simulink model "FM_Broadcast_CE2251"  (R2025a)
settings: Solver=FixedStepDiscrete  StartTime=0.0  StopTime=inf  RelTol=1e-3  EnableMultiTasking=on
PostLoadFcn:
  | blk = [gcs,'/Spectrum Analyzer'];
  | cfg = get_param(blk,'ScopeConfiguration');
libraries: dspsnks4 x1, dspsigops x1, commanabbnd3 x1, sdrrlib x1
CloseFcn:
  | clear blk cfg cf dialParam GetMaskObj maxCF minCF tune_cmd;
settings Model: Creator=The MathWorks, Inc.  LastModifiedBy=mthom
settings SolverCC: AlgebraicLoopSolver=TrustRegion
settings DataIOCC: LimitDataPoints=on  SaveFormat=Array  SaveOutput=off  SignalLogging=off  DSMLogging=off  SaveTime=off  ReturnWorkspaceOutputs=off
settings OptimizationCC: ExpressionDepthLimit=2147483647.0  LifeSpan=inf
settings DebuggingCC: UnderspecifiedInitializationDetection=Classic  MergeDetectMultiDrivingBlocksExec=none  SolverPrmCheckMsg=warning  ParameterPrecisionLossMsg=none  FcnCallInpInsideContextMsg=warning  UnconnectedInputMsg=warning  UnconnectedOutputMsg=warning  UnconnectedLineMsg=warning  AllowSymbolicDim=off  StateNameClashWarn=warning  SFUnexpectedBacktrackingDiag=warning  SFNoUnconditionalDefaultTransitionDiag=warning  SFExecutionAtInitializationDiag=none  ArithmeticOperatorsInVariantConditions=warning
settings HardwareCC: ProdBitPerPointer=32.0  ProdBitPerSizeT=32.0  ProdBitPerPtrDiffT=32.0  ProdLargestAtomicFloat=None  ProdIntDivRoundTo=Undefined  ProdEndianess=Unspecified  ProdWordSize=32.0  ProdHWDeviceType=32-bit Generic  TargetBitPerPointer=64.0  TargetBitPerSizeT=64.0  TargetBitPerPtrDiffT=64.0  TargetLongLongMode=on  TargetIntDivRoundTo=Zero  TargetEndianess=LittleEndian  TargetWordSize=64.0  TargetHWDeviceType=Generic->MATLAB Host Computer  ProdEqTarget=off
settings ModelReferenceCC: EnableRefExpFcnMdlSchedulingChecks=on  PropagateSignalLabelsOutOfModel=off
settings SFSimCC: SimUseLocalCustomCode=off  CustomCodeUndefinedFunction=UseInterfaceOnly
settings RTWCC: RTWUseLocalCustomCode=off  GPUComputeCapability=3.5
settings RTWCC: CustomSourceCode=|
  | #include<stdio.h>
  | #include<stdlib.h>
settings CodeAppCC: StateflowObjectComments=on
settings GRTTargetCC: TargetLangStandard=C89/C90 (ANSI)  CombineOutputUpdateFcns=off  GRTInterface=on
settings ConfigComp: CovMetricSettings=dw  CovSaveCumulativeToWorkspaceVar=on  CovSaveSingleToWorkspaceVar=on  CovExternalEMLEnable=off  CovSFcnEnable=off

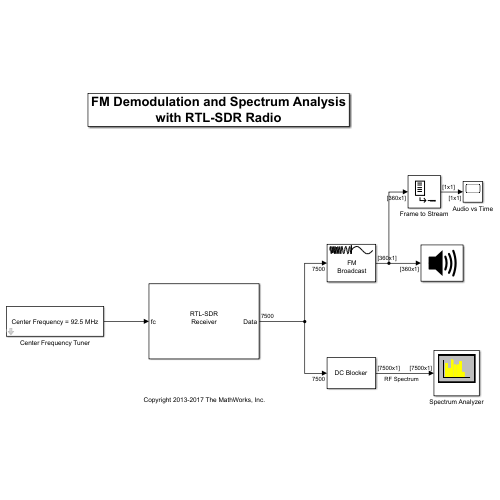
[thumbnail: Simulink's stored preview of the top-level diagram]
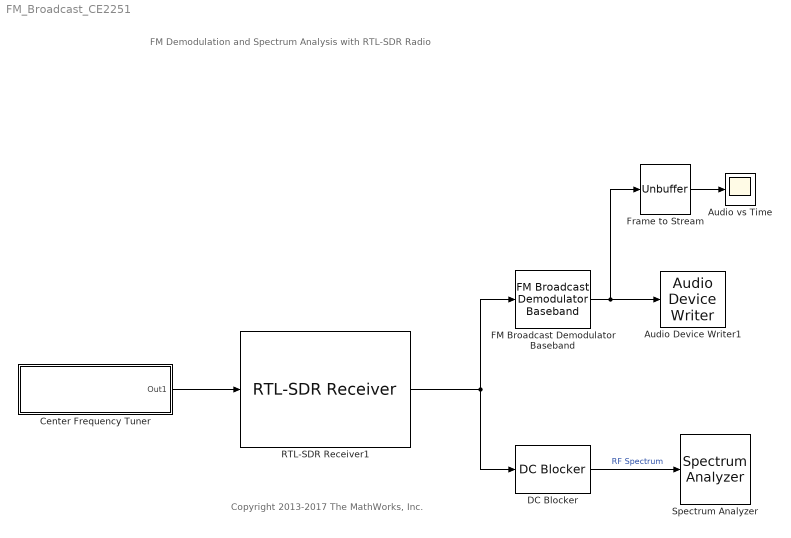
== system FM_Broadcast_CE2251 ==
  note: FM Demodulation and Spectrum Analysis
      | with RTL-SDR Radio
  note: Copyright 2013-2017 The MathWorks, Inc.
  Audio Device Writer1 : dspsnks4/Audio Device Writer  Driver=DirectSound  Device=Default  InheritSampleRate=on  SampleRate=44100  BitDepth=16-bit integer  BufferSize=4096  NumBuffers=10  DefaultOutputChannelMapping=on  OutputChannelMapping=1:2  OutputNumUnderrunSamples=off  DriverIdx=1  DeviceWarnFlag=''
  Audio vs Time : Scope
      settings: TimeSpan=100e-3  ActiveDisplayYMinimum=-0.55658585126871019  ActiveDisplayYMaximum=0.60385066284171973
  Center Frequency Tuner : Subsystem  mask{CenterFrequency=92.5, MinCenterFrequency=87.7, MaxCenterFrequency=107.9}
      mask prompts: CenterFrequency "Center Frequency (MHz)"; MinCenterFrequency "Min Center Frequency (MHZ)"; MaxCenterFrequency "Max Center Frequency (MHz)"
      mask Callback CenterFrequency:
      | % Get the center frequency value from the center frequency tuner
      | cf = str2num(get_param(gcb,'CenterFrequency'));
      | if isempty(cf)
      |     % Default Value
      |     cf = 102.5;
      | end
      | cf = cf.*1e6;
      | % Tune command used to set the Frequency offset on the spectrum analyzer
      | tune_cmd = ['cfg.FrequencyOffset = ''' num2str(cf) ''';'];
      | % Evaluate the tuning command in the base workspace
      | evalin('base',tune_cmd);
      mask Callback MinCenterFrequency:
      | GetMaskObj = Simulink.Mask.get(gcb);
      | dialParam = GetMaskObj.getParameter('CenterFrequency');
      | minCF = get_param(gcb,'MinCenterFrequency');
      | maxCF = get_param(gcb,'MaxCenterFrequency');
      | if isempty(minCF)
      |     minCF = 87.7;
      | end
      | if isempty(maxCF)
      |    macCF = 107.9;
      | end
      | 
      | if ~isempty(minCF) && ~isempty(maxCF)
      |  try
      |     dialParam.Range = [str2num(minCF),str2num(maxCF)];
      |  catch
      |  end
      | end
      mask Callback MaxCenterFrequency:
      | GetMaskObj = Simulink.Mask.get(gcb);
      | dialParam = GetMaskObj.getParameter('CenterFrequency');
      | minCF = get_param(gcb,'MinCenterFrequency');
      | maxCF = get_param(gcb,'MaxCenterFrequency');
      | if isempty(minCF)
      |     minCF = 87.7;
      | end
      | if isempty(maxCF)
      |    macCF = 107.9;
      | end
      | 
      | if ~isempty(minCF) && ~isempty(maxCF)
      |  try
      |     dialParam.Range = [str2num(minCF),str2num(maxCF)];
      |  catch
      |  end
      | end
      mask DialogControl CenterFrequencyContainer Prompt: SDR Center Frequency (MHz)
      mask DialogControl FrequencyRangeContainer Prompt: Frequency Range (MHz)
      mask Display: fprintf('Center Frequency = %3.1f MHz',CenterFrequency);
  DC Blocker : dspsigops/DC Blocker  Algorithm=Subtract mean  NormalizedBandwidth=0.001  Length=50  Order=6  SimulateUsing=Code generation
  FM Broadcast Demodulator Baseband : commanabbnd3/FM Broadcast Demodulator Baseband  SampleRate=1e6  FrequencyDeviation=75e3  FilterTimeConstant=75e-6  AudioSampleRate=48000  PlaySound=off  BufferSize=5120  Stereo=off  RBDS=off  RBDSSamplesPerSymbol=10  RBDSCostasLoop=off  SimulateUsing=Interpreted execution
  Frame to Stream : Unbuffer
  RTL-SDR Receiver1 : sdrrlib/RTL-SDR Receiver  IPAddress=0  CenterFrequencySource=Input port  CenterFrequency=102.5e6  GainSource=AGC  Gain=0  ADCRate=1e6  FrequencyCorrection=0  LostSamplesOutputPort=off  LatencyOutputPort=off  OutputDataType=double  FrameLength=7500  EnableBurstMode=off  NumFramesInBurst=20  sobjType=sdrr.internal.SDRRTLReceiverSL  dataUDPPort=-1  ctrlUDPPort=-1  subDeviceList=nosubdev  sdrBlockType=SDRBlockTypeSLT.SDRRxBlock  requester=UNUSED_BY_SFCN  sdrExecutionMode=SDRExecutionModeSLT.ExecModeHW  BypassUserLogic=off  DecimatorSelect=DDC decimator  SourceSelect=RF data  SineAmplitude=16000  EnableInternalClock=off  BypassIQBalance=off  IFBandwidth=40e6  ADCRateSource=Dialog  IntermediateFrequency=0  DecimationFactorSource=Dialog  DecimationFactor=512  RFFrequencyIsTunable=logical(1)  SampleTime=(7500)/(1e6)  IFBandwidthSource=Dialog  SineFrequency=30000  BypassDCBlockingFilter=off  IntermediateFrequencySource=Dialog  IQBalanceCoefficients=64  SkipAllHardwareResetAndInitialization=off  EnableIQCalibrationTable=on  CacheIQCalibrationTable=off  EnableOffsetTuning=off  EnableRTLAGC=off  EnableTestMode=off  EnableTunerAGC=on  FrequencyCorrectionSource=Dialog  NumMLBuffers=128  NumUSBBuffers=16  RTLCrystalFrequency=28800000  TunerCrystalFrequency=28800000
  Spectrum Analyzer : SpectrumAnalyzer  Tag=simrfV2util1/Spectrum Analyzer  WindowPosition=[2002.000000,166.000000,820.000000,607.000000,]  Visible=on  ScopeFrameLocation=window  Method=Welch  Span=1000000  CenterFrequency=92500000  StartFrequency=92000000  StopFrequency=93000000  AveragingMethod=Exponential  FrequencyOffset=92500000  YLimits=[-41.5769 26.4856]  ColorLimits=[-36.0323 17.7815]  SelectedToolstripTab=spectrumAnalyzerToolstrip.channelMeasurementsTab  AllowFFTLengthLessThanSamplesPerUpdate=on
  wires:
  RTL-SDR Receiver1/1 -> FM Broadcast Demodulator Baseband/1, DC Blocker/1
  DC Blocker/1 -> Spectrum Analyzer/1  "RF Spectrum"
  Center Frequency Tuner/1(Out1) -> RTL-SDR Receiver1/1
  FM Broadcast Demodulator Baseband/1 -> Frame to Stream/1, Audio Device Writer1/1
  Frame to Stream/1 -> Audio vs Time/1

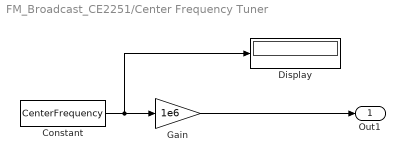
== system FM_Broadcast_CE2251/Center Frequency Tuner ==
  Constant : Constant  Value=CenterFrequency  SampleTime=-1
  Display : Display
  Gain : Gain  Gain=1e6
  Out1 : Outport  VectorParamsAs1DForOutWhenUnconnected=off
  wires:
  Constant/1 -> Display/1, Gain/1
  Gain/1 -> Out1/1
